simulink model "nucleo_f446re_Interrupt_push_button"  (R2015a)
settings: Solver=FixedStepDiscrete  SolverMode=SingleTasking  StartTime=0.0  StopTime=10.0  FixedStep=1e-3  RelTol=1e-3
libraries: mbed_targets_stm_nucleo_f446 x2, mbed_lib x1
settings Model: CovSFcnEnable=off  Creator=oh  LastModifiedBy=oh
settings OptimizationCC: OptimizeModelRefInitCode=on  LifeSpan=1
settings DebuggingCC: SolverPrmCheckMsg=warning
settings HardwareCC: ProdLargestAtomicInteger=Long  ProdLargestAtomicFloat=Double  ProdEndianess=LittleEndian  ProdHWDeviceType=ARM Compatible->ARM Cortex
settings RTWCC: SystemTargetFile=mbed.tlc  TemplateMakefile=mbed.tmf  Description=Mbed Target (Embedded Target)  TargetLang=C++
settings CodeAppCC: IgnoreCustomStorageClasses=off
settings STFCustomTargetCC: CombineOutputUpdateFcns=on  SupportContinuousTime=off  SupportVariableSizeSignals=off  SystemTargetFile=mbed.tlc
settings ERTTargetCC: SupportContinuousTime=off  SupportVariableSizeSignals=off  ERTCustomFileTemplate=mbed_file_process.tlc

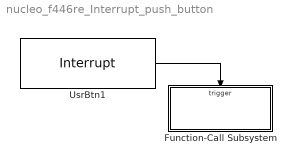
== system nucleo_f446re_Interrupt_push_button ==
  Function-Call Subsystem : Subsystem  TreatAsAtomicUnit=on
  UsrBtn1 : mbed_lib/GPIO/Interrupt  PortName=C  PinName=13  Interrupt=Both
  wires:
  UsrBtn1/1 -> Function-Call Subsystem/Trigger

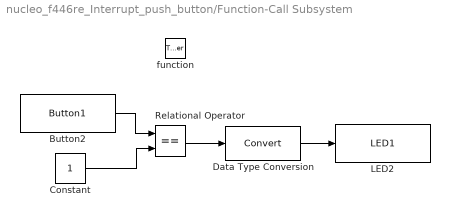
== system nucleo_f446re_Interrupt_push_button/Function-Call Subsystem ==
  function : TriggerPort  TriggerType=function-call
  Button2 : mbed_targets_stm_nucleo_f446/Button1  Parameter1=0
  Constant : Constant
  Data Type Conversion : DataTypeConversion
  LED2 : mbed_targets_stm_nucleo_f446/LED1  Parameter1=0
  Relational Operator : RelationalOperator  Operator===  OutDataTypeStr=boolean
  wires:
  Button2/1 -> Relational Operator/1
  Constant/1 -> Relational Operator/2
  Relational Operator/1 -> Data Type Conversion/1
  Data Type Conversion/1 -> LED2/1
